simulink library "AnomalyGeneratorLib"  (R2023b)
settings: Solver=VariableStepAuto  StartTime=0.0  StopTime=10.0  RelTol=1e-3
values from neighbouring files (symbols this model uses):
  DCSourceVoltageDrop = generateValues(DefaultModelParameters.DCSourceVoltageDrop,0.2,numSim, [0 inf])    [generateData.m]
  DCSourceVoltageDropDuration = generateValues(DefaultModelParameters.DCSourceVoltageDropDuration,0.2,numSim, [20 120])    [generateData.m]
undefined symbols (not defined in the file or in its folder): NumDCSourceAnomalies, SimEndTime
settings Model: Creator=astother  LastModifiedBy=anarasim
settings SolverCC: AlgebraicLoopSolver=TrustRegion
settings DebuggingCC: UnconnectedInputMsg=warning  UnconnectedOutputMsg=warning  UnconnectedLineMsg=warning
settings ModelReferenceCC: EnableRefExpFcnMdlSchedulingChecks=on
settings RTWCC: DLArmComputeVersion=19.05

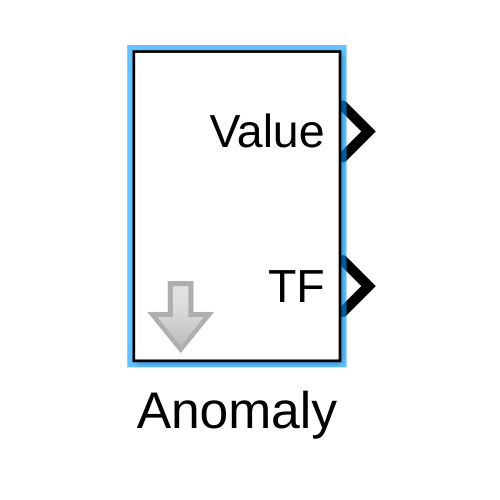
[thumbnail: Simulink's stored preview of the top-level diagram]
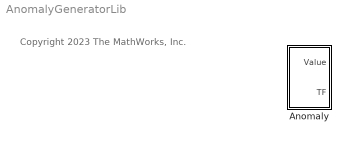
== system AnomalyGeneratorLib ==
  note: Copyright 2023 The MathWorks, Inc.
  Anomaly : Subsystem  mask{EndTime=SimEndTime, NumAnomalies=NumDCSourceAnomalies, AnomalyDuration=DCSourceVoltageDropDuration, AnomalyAmplitude=DCSourceVoltageDrop, RngSeed=0}
      mask prompts: EndTime "Time Window"; NumAnomalies "Num Anomalies"; AnomalyDuration "Anomaly Duration"; AnomalyAmplitude "Anomaly Amplitude"; RngSeed "Random Seed"

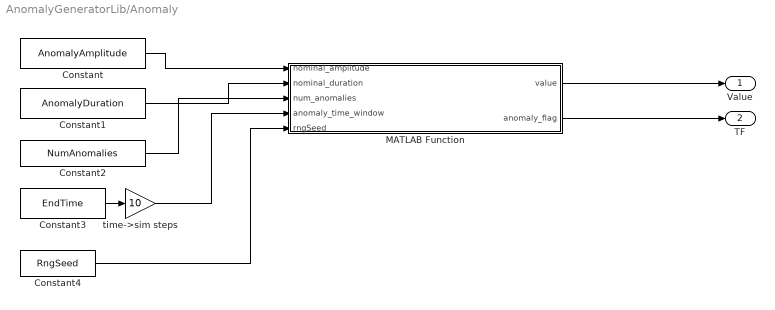
== system AnomalyGeneratorLib/Anomaly ==
  Constant : Constant  Value=AnomalyAmplitude
  Constant1 : Constant  Value=AnomalyDuration
  Constant2 : Constant  Value=NumAnomalies
  Constant3 : Constant  Value=EndTime
  Constant4 : Constant  Value=RngSeed
  MATLAB Function : MATLAB Function  TreatAsAtomicUnit=on
  time->sim steps : Gain  Gain=10
  Value : Outport
  TF : Outport  Port=2
  wires:
  MATLAB Function/2(anomaly_flag) -> TF/1
  time->sim steps/1 -> MATLAB Function/4(anomaly_time_window)
  Constant4/1 -> MATLAB Function/5(rngSeed)
  Constant3/1 -> time->sim steps/1
  Constant2/1 -> MATLAB Function/3(num_anomalies)
  Constant1/1 -> MATLAB Function/2(nominal_duration)
  Constant/1 -> MATLAB Function/1(nominal_amplitude)
  MATLAB Function/1(value) -> Value/1

== matlab function AnomalyGeneratorLib/Anomaly/MATLAB Function ==
  data: nominal_amplitude input; nominal_duration input; value output; num_anomalies input; anomaly_time_window input; anomaly_flag output; rngSeed input
function [value,anomaly_flag]  = fcn(nominal_amplitude,nominal_duration,num_anomalies,anomaly_time_window,rngSeed)

persistent flag
persistent running_duration
persistent duration
persistent anomaly_count
persistent amplitude
persistent ticks
persistent startpoints

if isempty(flag)
    flag = false;
    rng(rngSeed);
    startpoints = sort(randperm(anomaly_time_window,num_anomalies));
    anomaly_count = 1;
end
if isempty(running_duration)
    running_duration = 0;
end
if isempty(duration)
    duration = 0;
end
if isempty(amplitude)
    amplitude = nominal_amplitude;
end
if isempty(ticks)
    ticks = 0;
end

if flag && running_duration < duration
    flag = true;
    running_duration = running_duration+1;
    value = amplitude;
else
    flag = false;
    running_duration = 0;
    value = 0;
    %Do we want to enable?
    if lTriggerAnomaly(anomaly_count,startpoints,ticks)
        anomaly_count = anomaly_count + 1;
        duration = nominal_duration + (0.2*nominal_duration)^2*rand(1);
        amplitude = nominal_amplitude + (0.2*nominal_amplitude)^2*rand(1);
        running_duration = 0;
        %disp("Anomaly: (" + duration + ", " + amplitude + ")");
        flag = true;
    end
end
if ticks <= anomaly_time_window
    ticks = ticks+1;
else
    ticks = 0;
    startpoints = sort(randperm(anomaly_time_window,num_anomalies));
    anomaly_count = 1;
end

anomaly_flag = flag;
end

function tf = lTriggerAnomaly(anomaly_count,startpoints,ticks)

tf = numel(startpoints) >= anomaly_count && ticks > startpoints(anomaly_count);
end
